simulink model "Frame"  (R2021b)
settings: Solver=ode3  StartTime=0.0  StopTime=10  FixedStep=Ts  RelTol=1e-3
model workspace (MAT data in the model file):
  Ts = 0.005
libraries: visionfilter x1, simulink x1, cstblocks x1
settings Model: Creator=GUBED49  LastModifiedBy=merciegu

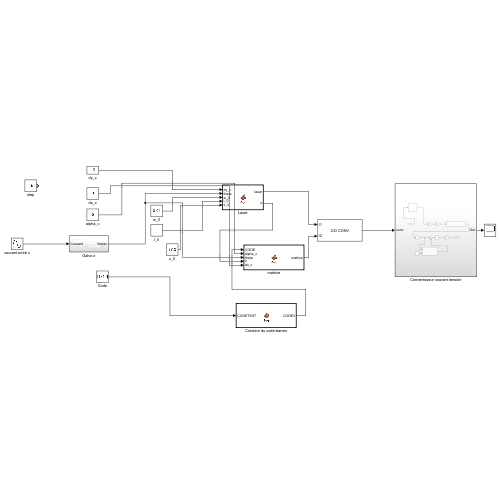
[thumbnail: Simulink's stored preview of the top-level diagram]
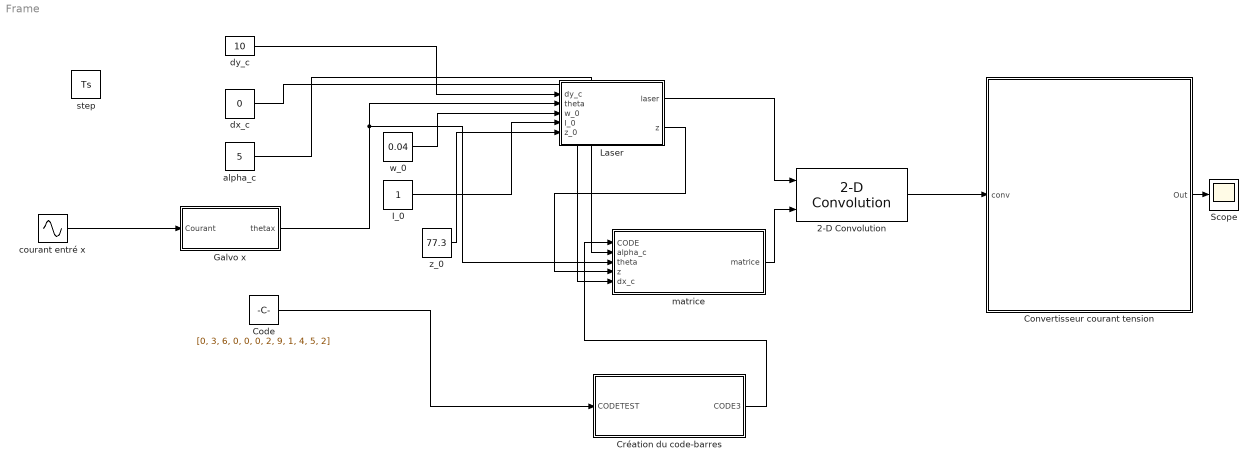
== system Frame ==
  2-D Convolution : visionfilter/2-D Convolution  outSize=Full  normalize=off  roundingMode=Floor  overflowMode=off  prodOutputMode=Binary point scaling  prodOutputWordLength=32  prodOutputFracLength=10  outputMode=Binary point scaling  outputWordLength=32  outputFracLength=12
      settings: SourceProductBaseCode=VP
  Code : Constant  Value=[0, 3, 6, 0, 0, 0, 2, 9, 1, 4, 5, 2]
  Convertisseur courant tension : Subsystem
  Création du code-barres : MATLAB Function  TreatAsAtomicUnit=on
  Galvo x : Subsystem
  I_0 : Constant
  Laser : MATLAB Function  TreatAsAtomicUnit=on
  Scope : Scope
  alpha_c : Constant  Value=5
  courant entré x : Sin  Amplitude=180  SampleTime=0
  dx_c : Constant  Value=0
  dy_c : Constant  Value=10
  matrice : MATLAB Function  TreatAsAtomicUnit=on
  step : Constant  Value=Ts
  w_0 : Constant  Value=0.04
  z_0 : Constant  Value=77.3
  wires:
  Code/1 -> Création du code-barres/1(CODETEST)
  dy_c/1 -> Laser/1(dy_c)
  Galvo x/1(" thetax") -> matrice/3(theta), Laser/2(theta)
  w_0/1 -> Laser/3(w_0)
  I_0/1 -> Laser/4(I_0)
  z_0/1 -> Laser/5(z_0)
  Création du code-barres/1(CODE3) -> matrice/1(CODE)
  alpha_c/1 -> matrice/2(alpha_c)
  Laser/2(z) -> matrice/4(z)
  dx_c/1 -> matrice/5(dx_c)
  matrice/1(matrice) -> 2-D Convolution/2
  Laser/1(laser) -> 2-D Convolution/1
  courant entré x/1 -> Galvo x/1(Courant)
  2-D Convolution/1 -> Convertisseur courant tension/1(conv)
  Convertisseur courant tension/1(Out) -> Scope/1

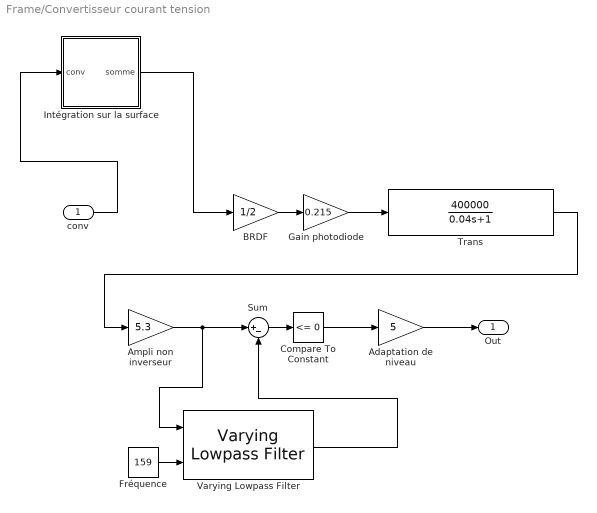
== system Frame/Convertisseur courant tension ==
  conv : Inport
  Adaptation de niveau : Gain  Gain=5
  Ampli non inverseur : Gain  Gain=5.3
  BRDF : Gain  Gain=1/2
  Compare To Constant : simulink/Logic and Bit Operations/Compare To Constant  relop=<=  const=0  OutDataTypeStr=boolean
  Fréquence : Constant  Value=159
  Gain photodiode : Gain  Gain=0.215
  Intégration sur la surface : MATLAB Function  TreatAsAtomicUnit=on
  Sum : Sum  Inputs=|+-
  Trans : TransferFcn  Numerator=[400000]  Denominator=[0.04,1]
  Varying Lowpass Filter : cstblocks/Linear Parameter Varying/Varying Lowpass Filter  N=1
  Out : Outport
  wires:
  Fréquence/1 -> Varying Lowpass Filter/2
  Trans/1 -> Ampli non inverseur/1
  Sum/1 -> Compare To Constant/1
  Intégration sur la surface/1(somme) -> BRDF/1
  Ampli non inverseur/1 -> Varying Lowpass Filter/1, Sum/1
  BRDF/1 -> Gain photodiode/1
  Gain photodiode/1 -> Trans/1
  Varying Lowpass Filter/1 -> Sum/2
  Adaptation de niveau/1 -> Out/1
  Compare To Constant/1 -> Adaptation de niveau/1
  conv/1 -> Intégration sur la surface/1(conv)

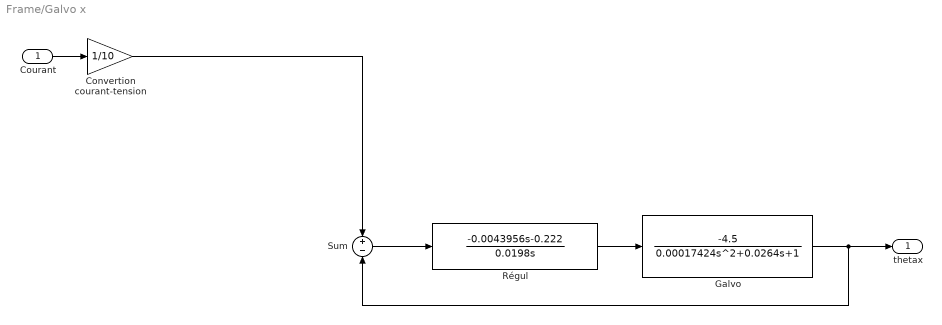
== system Frame/Galvo x ==
  Courant : Inport
  Convertion courant-tension : Gain  Gain=1/10
  "Galvo " : TransferFcn  Numerator=[-4.5]  Denominator="[0.00017424, 0.0264  1]"
  Régul : TransferFcn  Numerator=[-0.0043956, -0.222]  Denominator=[0.0198,0]
  Sum : Sum  Inputs=+|-
  " thetax" : Outport
  wires:
  Courant/1 -> Convertion courant-tension/1
  Convertion courant-tension/1 -> Sum/1
  Sum/1 -> Régul/1
  "Galvo "/1 -> " thetax"/1, Sum/2
  Régul/1 -> "Galvo "/1

== matlab function Frame/Laser ==
  data: dy_c input; laser output; theta input; w_0 input; I_0 input; z_0 input; z output
function [laser, z] = fcn(dy_c, theta, w_0, I_0, z_0)

z=dy_c/cosd(theta+0.000000000001);
w = (w_0*sqrt(1+(z/z_0)^2));
pas=0.33;
laser4=zeros(5,5);
for col= 1 : 5
    for row = 1 : 5
        col_1= (col*pas)-pas;
        row_1= (row*pas)-pas;
        rayon=sqrt(row_1^2+col_1^2);
laser4(row, col) = (I_0*(w_0/w)^(2)*exp((-2*((rayon)^2))/(w^2)));

    end
end
laser3=fliplr(laser4);
laser1=flipud(laser4);
laser2=fliplr(laser1);
laser=[laser2 laser1; laser3 laser4];

== matlab function Frame/Création du code-barres ==
  data: CODETEST input; CODE3 output
function CODE3 = fcn(CODETEST)


GAUCHE = [0 0 0 1 1 0 1; 0 0 1 1 0 0 1; 0 0 1 0 0 1 1; 0 1 1 1 1 0 1; 0 1 0 0 0 1 1; 0 1 1 0 0 0 1; 0 1 0 1 1 1 1; 0 1 1 1 0 1 1; 0 1 1 0 1 1 1; 0 0 0 1 0 1 1];
DROITE = [1 1 0 0 1 1 0; 1 1 0 1 1 0 0; 1 0 0 0 0 1 0; 1 0 1 1 1 0 0; 1 0 0 1 1 1 0; 1 0 1 0 0 0 0; 1 0 0 0 1 0 0; 1 0 0 1 0 0 0; 1 1 1 0 1 0 0; 1 1 1 0 0 1 0];



%Génération du code-barres

START=[ 1 0 1];
END=[1 0 1];
MIDDLE=[0 1 0 1 0];
QUIET=zeros(1,9);
CGAUCHE=[];
CDROITE=[];

for i = 1: 6
    val=CODETEST(i);
    val=val+1;
    CGAUCHE = [CGAUCHE,GAUCHE(val,:)];
end

for j = 7 : 12
    val=CODETEST(j);
    val=val+1;
    CDROITE = [CDROITE, DROITE(val, :)];
end 

CGAUCHE=transpose(CGAUCHE);
CDROITE=transpose(CDROITE);
CGAUCHE=reshape(CGAUCHE,1,42);
CDROITE=reshape(CDROITE,1,42);
CODE=[ QUIET START CGAUCHE MIDDLE CDROITE END QUIET];
CODEBAS= [ QUIET START zeros([1 42]) MIDDLE zeros([1 42]) END QUIET];


for i=1:(77)
    CODE2=[CODE;CODE(1,:)];
end
for i=1:(5)
    CODE3=[CODE2;CODEBAS(1,:)];
end

== matlab function Frame/Convertisseur courant tension/Intégration sur la surface ==
  data: conv input; somme output
function somme = fcn(conv)
somme=sum(sum(conv(:)));

== matlab function Frame/matrice ==
  data: CODE input; matrice output; alpha_c input; theta input; z input; dx_c input
function matrice  = fcn(CODE, alpha_c, theta,z, dx_c)
x =(sind(theta+0.00000000001)*z)-dx_c ;
c = round((x/cosd(alpha_c))/0.033);
if c < -53
c=-53;
end
if c > 53
    c=53;
end
    
matrice=CODE(:, 54+c);
